simulink model "sim_Pendulum_hangingFromHarmonicOscillator"  (R2020a)
settings: Solver=VariableStepAuto  StartTime=0.0  StopTime=t_sim  MaxStep=0.1  RelTol=1e-3
values from neighbouring files (symbols this model uses):
  g = 9.8    [Pendulum_hangingFromHarmonicOscillator.m]    (also in Pendulum_withFreeSupport.m)
  k = 20    [MSDSystem_eg2.m]    (also in Pendulum_hangingFromHarmonicOscillator.m)
  L = 10    [Pendulum_hangingFromHarmonicOscillator.m]
  M = feedback(Gc*Gp, H)    [MSDSystem_eg2.m]    (also in Pendulum_hangingFromHarmonicOscillator.m = 400; Pendulum_withFreeSupport.m = 400)
  m = 10    [MSDSystem_eg1.m]    (also in MSDSystem_eg2.m = 4; Pendulum_hangingFromHarmonicOscillator.m = 200; Pendulum_withFreeSupport.m = 200)
  theta0_rad = (pi/180)*theta0    (= 0.523598775598)    [Pendulum_hangingFromHarmonicOscillator.m]    (also in Pendulum_withFreeSupport.m)
  v0 = 6    [Pendulum_hangingFromHarmonicOscillator.m]    (also in Pendulum_withFreeSupport.m)
settings Model: Creator=Samir  LastModifiedBy=Samir

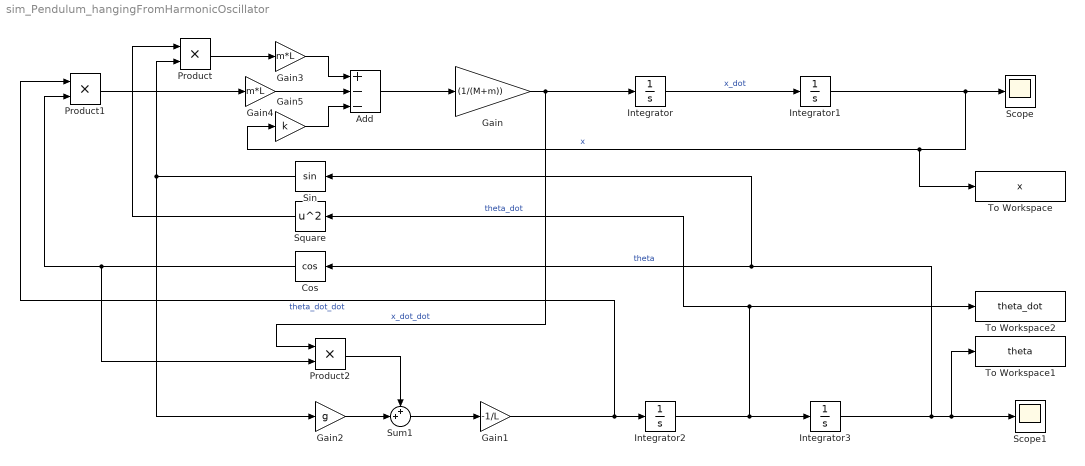
== system sim_Pendulum_hangingFromHarmonicOscillator ==
  Add : Sum  Inputs=+--
  Cos : Trigonometry  Operator=cos
  Gain : Gain  Gain=(1/(M+m))
  Gain1 : Gain  Gain=-1/L
  Gain2 : Gain  Gain=g
  Gain3 : Gain  Gain=m*L
  Gain4 : Gain  Gain=m*L
  Gain5 : Gain  Gain=k
  Integrator : Integrator  InitialCondition=v0
  Integrator1 : Integrator
  Integrator2 : Integrator
  Integrator3 : Integrator  InitialCondition=theta0_rad
  Product : Product
  Product1 : Product
  Product2 : Product
  Scope : Scope
  Scope1 : Scope
  Sin : Trigonometry
  Square : Math  Operator=square  SaturateOnIntegerOverflow=on
  Sum1 : Sum  Inputs=++|
  To Workspace : ToWorkspace  VariableName=x  SaveFormat=Timeseries  SampleTime=-1
  To Workspace1 : ToWorkspace  VariableName=theta  SaveFormat=Timeseries  SampleTime=-1
  To Workspace2 : ToWorkspace  VariableName=theta_dot  SaveFormat=Timeseries  SampleTime=-1
  wires:
  Integrator/1 -> Integrator1/1  "x_dot"
  Integrator1/1 -> Gain5/1, To Workspace/1, Scope/1  "x"
  Gain/1 -> Product2/1, Integrator/1  "x_dot_dot"
  Gain1/1 -> Product1/1, Integrator2/1  "theta_dot_dot"
  Integrator3/1 -> Cos/1, Sin/1, Scope1/1, To Workspace1/1  "theta"
  Integrator2/1 -> To Workspace2/1, Square/1, Integrator3/1  "theta_dot"
  Square/1 -> Product/1
  Sin/1 -> Gain2/1, Product/2
  Cos/1 -> Product2/2, Product1/2
  Sum1/1 -> Gain1/1
  Gain2/1 -> Sum1/2
  Product2/1 -> Sum1/1
  Add/1 -> Gain/1
  Gain3/1 -> Add/1
  Product/1 -> Gain3/1
  Gain4/1 -> Add/2
  Product1/1 -> Gain4/1
  Gain5/1 -> Add/3
